simulink model "Vehicle_Radar_Model"  (R2013a)
settings: Solver=ode4  StartTime=0.0  StopTime=100  FixedStep=0.001  MaxStep=0.001  RelTol=1e-3
model workspace (MAT data in the model file):
  m = 1530
  lf = 1.11
  lr = 1.6662
  R_Tire = 0.33
  Iyy_Tire = 0.9
  Pb2Tq_f = 300
  Pb2Tq_r = 150
  Fx_SL = [-1; -0.9; -0.8; -0.7; -0.6; -0.5; -0.4; -0.3; -0.25; -0.2; -0.18; -0.16; -0.14; -0.12; -0.1; -0.08; -0.06; -0.04; -0.02; 0; 0.02; 0.04; 0.06; 0.08; 0.1; 0.12; 0.14; 0.16; 0.18; 0.2; 0.25; 0.3; 0.4; 0.5; 0.6; 0.7; 0.8; 0.9; 1]
  Fx_W = [2105 3995 6120 7900 10100]
  Fx_Data = [-2029.26  -4058.51  -6087.76  -8117.01  -10146.3; -2029.26  -4058.51  -6087.76  -8117.01  -10146.3; -2053.55  -4107.12  -6160.67  -8214.24  -10267.8; -2084.58  -4169.16  -6253.75  -8338.33  -10422.9; -2125.47  -4250.95  -6376.42  -8501.91  -10627.4; -2181.64  -4363.28  -6544.93  -8726.56  -10908.2; -2262.94  -4525.87  -6788.82  -9051.76  -11314.7; -2388.22  -4776.46  -7164.69  -9552.92  -11941.1; -2476.95  -4953.9  -7430.85  -9907.79  -12384.7; -2586.89  -5173.78  -7760.68  -10347.6  -12934.4; -2634.75  -5269.5  -7904.24  -10539  -13173.7; -2680.7  -5361.4  -8042.1  -10722.8  -13403.5; -2717.36  -5434.73  -8152.09  -10869.4  -13586.8; -2729.82  -5459.63  -8189.45  -10919.3  -13649.1; -2689.78  -5379.54  -8069.32  -10759.1  -13448.8; -2548.95  -5097.92  -7646.88  -10195.8  -12744.8; -2240.07  -4480.13  -6720.21  -8960.27  -11200.3; -1701.43  -3402.86  -5104.29  -6805.72  -8507.15; -926.741  -1853.48  -2780.22  -3706.97  -4633.7; 0  0  0  0  0; 926.741  1853.48  2780.22  3706.97  4633.7; 1701.43  3402.86  5104.29  6805.72  8507.15; 2240.07  4480.13  6720.21  8960.27  11200.3; 2548.95  5097.92  7646.88  10195.8  12744.8; 2689.78  5379.54  8069.32  10759.1  13448.8; 2729.82  5459.63  8189.45  10919.3  13649.1; 2717.36  5434.73  8152.09  10869.4  13586.8; 2680.7  5361.4  8042.1  10722.8  13403.5; 2634.75  5269.5  7904.24  10539  13173.7; 2586.89  5173.78  7760.68  10347.6  12934.4; 2476.95  4953.9  7430.85  9907.79  12384.7; 2388.22  4776.46  7164.69  9552.92  11941.1; 2262.94  4525.87  6788.82  9051.76  11314.7; 2181.64  4363.28  6544.93  8726.56  10908.2; 2125.47  4250.95  6376.42  8501.91  10627.4; 2084.58  4169.16  6253.75  8338.33  10422.9; 2053.55  4107.12  6160.67  8214.24  10267.8; 2029.26  4058.51  6087.76  8117.01  10146.3; 2029.26  4058.51  6087.76  8117.01  10146.3]
  g = 9.81
  l = 2.77622
  t2e = 2000
settings Model: Creator=Park  LastModifiedBy=IVDL
settings DataIOCC: LimitDataPoints=off  SignalLoggingSaveFormat=ModelDataLogs
settings OptimizationCC: ExpressionDepthLimit=2147483647
settings DebuggingCC: MultiTaskDSMMsg=warning  MultiTaskCondExecSysMsg=none  FcnCallInpInsideContextMsg=UseLocalSettings  StrictBusMsg=None
settings RTWCC: IncludeERTFirstTime=on
settings GRTTargetCC: CodeReplacementLibrary=None  CombineOutputUpdateFcns=off  CPPClassGenCompliant=on  GRTInterface=on

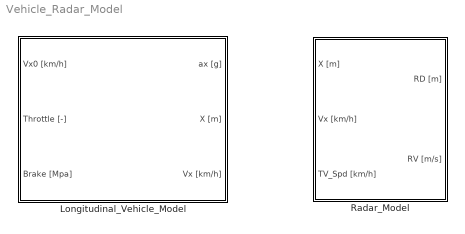
== system Vehicle_Radar_Model ==
  Longitudinal_Vehicle_Model : Subsystem
  Radar_Model : Subsystem

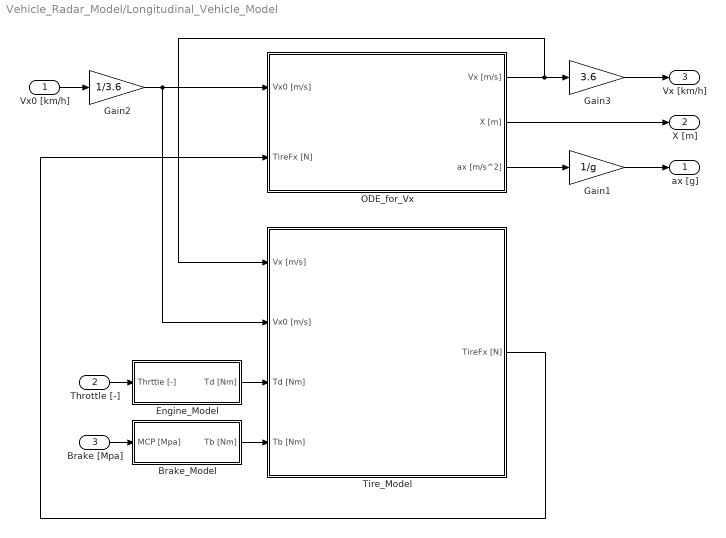
== system Vehicle_Radar_Model/Longitudinal_Vehicle_Model ==
  Vx0 [km/h] : Inport
  Throttle [-] : Inport  Port=2
  Brake [Mpa] : Inport  Port=3
  Brake_Model : Subsystem
  Engine_Model : Subsystem
  Gain1 : Gain  Gain=1/g
  Gain2 : Gain  Gain=1/3.6
  Gain3 : Gain  Gain=3.6
  ODE_for_Vx : Subsystem
  Tire_Model : Subsystem
  ax [g] : Outport
  X [m] : Outport  Port=2
  Vx [km/h] : Outport  Port=3
  wires:
  ODE_for_Vx/2(X [m]) -> X [m]/1
  Vx0 [km/h]/1 -> Gain2/1
  Engine_Model/1(Td [Nm]) -> Tire_Model/3(Td [Nm])
  Brake_Model/1(Tb [Nm]) -> Tire_Model/4(Tb [Nm])
  Brake [Mpa]/1 -> Brake_Model/1(MCP [Mpa])
  Throttle [-]/1 -> Engine_Model/1(Thrttle [-])
  Tire_Model/1(TireFx [N]) -> ODE_for_Vx/2(TireFx [N])
  ODE_for_Vx/3(ax [m/s^2]) -> Gain1/1
  Gain1/1 -> ax [g]/1
  ODE_for_Vx/1(Vx [m/s]) -> Gain3/1, Tire_Model/1(Vx [m/s])
  Gain2/1 -> ODE_for_Vx/1(Vx0 [m/s]), Tire_Model/2(Vx0 [m/s])
  Gain3/1 -> Vx [km/h]/1

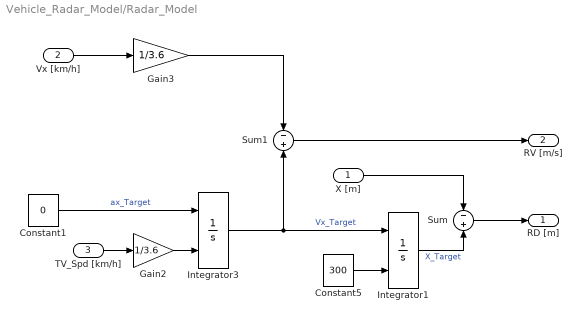
== system Vehicle_Radar_Model/Radar_Model ==
  X [m] : Inport
  Vx [km/h] : Inport  Port=2
  TV_Spd [km/h] : Inport  Port=3
  Constant1 : Constant  Value=0
  Constant5 : Constant  Value=300
  Gain2 : Gain  Gain=1/3.6
  Gain3 : Gain  Gain=1/3.6
  Integrator1 : Integrator  InitialConditionSource=external  InitialCondition=500
  Integrator3 : Integrator  InitialConditionSource=external  InitialCondition=80  LimitOutput=on  LowerSaturationLimit=0
  Sum : Sum  Inputs=-+
  Sum1 : Sum  Inputs=-+
  RD [m] : Outport
  RV [m/s] : Outport  Port=2
  wires:
  TV_Spd [km/h]/1 -> Gain2/1
  Constant1/1 -> Integrator3/1  "ax_Target"
  Integrator3/1 -> Integrator1/1, Sum1/2  "Vx_Target"
  Integrator1/1 -> Sum/2  "X_Target"
  Constant5/1 -> Integrator1/2
  Sum/1 -> RD [m]/1
  X [m]/1 -> Sum/1
  Vx [km/h]/1 -> Gain3/1
  Sum1/1 -> RV [m/s]/1
  Gain2/1 -> Integrator3/2
  Gain3/1 -> Sum1/1

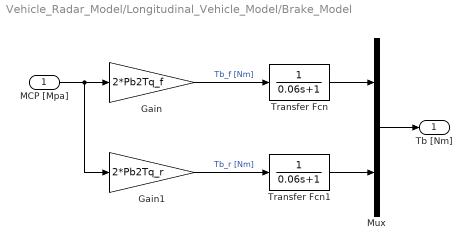
== system Vehicle_Radar_Model/Longitudinal_Vehicle_Model/Brake_Model ==
  MCP [Mpa] : Inport
  Gain : Gain  Gain=2*Pb2Tq_f
  Gain1 : Gain  Gain=2*Pb2Tq_r
  Mux : Mux  Inputs=2
  Transfer Fcn : TransferFcn  Denominator=[0.06 1]
  Transfer Fcn1 : TransferFcn  Denominator=[0.06 1]
  Tb [Nm] : Outport
  wires:
  Gain/1 -> Transfer Fcn/1  "Tb_f [Nm]"
  Gain1/1 -> Transfer Fcn1/1  "Tb_r [Nm]"
  MCP [Mpa]/1 -> Gain1/1, Gain/1
  Mux/1 -> Tb [Nm]/1
  Transfer Fcn/1 -> Mux/1
  Transfer Fcn1/1 -> Mux/2

== system Vehicle_Radar_Model/Longitudinal_Vehicle_Model/Engine_Model ==
  Thrttle [-] : Inport
  Gain : Gain  Gain=t2e
  Transfer Fcn : TransferFcn  Numerator=[100]  Denominator=[1 2*0.5*10 100]
  Td [Nm] : Outport
  wires:
  Thrttle [-]/1 -> Gain/1
  Gain/1 -> Transfer Fcn/1
  Transfer Fcn/1 -> Td [Nm]/1

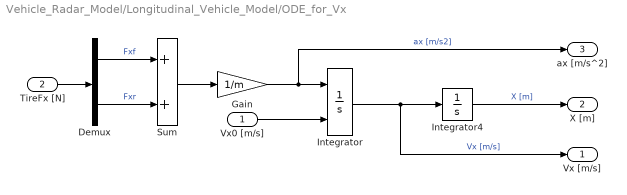
== system Vehicle_Radar_Model/Longitudinal_Vehicle_Model/ODE_for_Vx ==
  Vx0 [m/s] : Inport
  TireFx [N] : Inport  Port=2
  Demux : Demux  Outputs=2
  Gain : Gain  Gain=1/m
  Integrator : Integrator  InitialConditionSource=external
  Integrator4 : Integrator
  Sum : Sum
  Vx [m/s] : Outport
  X [m] : Outport  Port=2
  ax [m/s^2] : Outport  Port=3
  wires:
  Integrator4/1 -> X [m]/1  "X [m]"
  Vx0 [m/s]/1 -> Integrator/2
  Integrator/1 -> Integrator4/1, Vx [m/s]/1  "Vx [m/s]"
  Sum/1 -> Gain/1
  Gain/1 -> Integrator/1, ax [m/s^2]/1  "ax [m/s2]"
  TireFx [N]/1 -> Demux/1
  Demux/1 -> Sum/1  "Fxf"
  Demux/2 -> Sum/2  "Fxr"

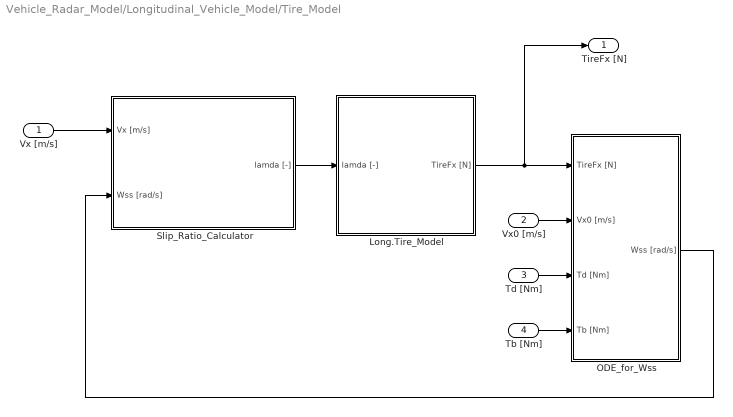
== system Vehicle_Radar_Model/Longitudinal_Vehicle_Model/Tire_Model ==
  Vx [m/s] : Inport
  Vx0 [m/s] : Inport  Port=2
  Td [Nm] : Inport  Port=3
  Tb [Nm] : Inport  Port=4
  Long.Tire_Model : Subsystem
  ODE_for_Wss : Subsystem
  Slip_Ratio_Calculator : Subsystem
  TireFx [N] : Outport
  wires:
  Long.Tire_Model/1(TireFx [N]) -> TireFx [N]/1, ODE_for_Wss/1(TireFx [N])
  Slip_Ratio_Calculator/1(lamda [-]) -> Long.Tire_Model/1(lamda [-])
  Vx [m/s]/1 -> Slip_Ratio_Calculator/1(Vx [m/s])
  Vx0 [m/s]/1 -> ODE_for_Wss/2(Vx0 [m/s])
  Td [Nm]/1 -> ODE_for_Wss/3(Td [Nm])
  Tb [Nm]/1 -> ODE_for_Wss/4(Tb [Nm])
  ODE_for_Wss/1(Wss [rad/s]) -> Slip_Ratio_Calculator/2(Wss [rad/s])

== system Vehicle_Radar_Model/Longitudinal_Vehicle_Model/Tire_Model/Long.Tire_Model ==
  lamda [-] : Inport
  Demux : Demux  Outputs=2
  Fx_f_Calculator : Subsystem
  Fx_r_Calculator : Subsystem
  Mux : Mux  Inputs=2
  TireFx [N] : Outport
  wires:
  lamda [-]/1 -> Demux/1
  Demux/1 -> Fx_f_Calculator/1(lamda_f [-])
  Demux/2 -> Fx_r_Calculator/1(lamda_r [-])
  Fx_f_Calculator/1(TireFx _f [N]) -> Mux/1
  Fx_r_Calculator/1(TireFx _r [N]) -> Mux/2
  Mux/1 -> TireFx [N]/1

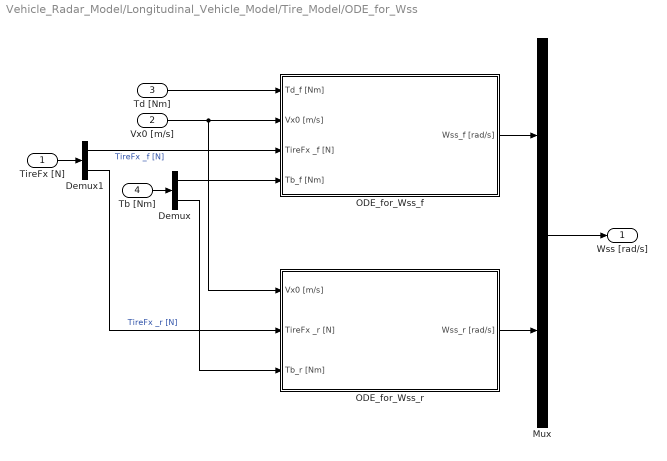
== system Vehicle_Radar_Model/Longitudinal_Vehicle_Model/Tire_Model/ODE_for_Wss ==
  TireFx [N] : Inport
  Vx0 [m/s] : Inport  Port=2
  Td [Nm] : Inport  Port=3
  Tb [Nm] : Inport  Port=4
  Demux : Demux  Outputs=2
  Demux1 : Demux  Outputs=2
  Mux : Mux  Inputs=2
  ODE_for_Wss_f : Subsystem
  ODE_for_Wss_r : Subsystem
  Wss [rad/s] : Outport
  wires:
  Demux1/1 -> ODE_for_Wss_f/3(TireFx _f [N])  "TireFx _f [N]"
  Td [Nm]/1 -> ODE_for_Wss_f/1(Td_f [Nm])
  Vx0 [m/s]/1 -> ODE_for_Wss_r/1(Vx0 [m/s]), ODE_for_Wss_f/2(Vx0 [m/s])
  Tb [Nm]/1 -> Demux/1
  Demux/1 -> ODE_for_Wss_f/4(Tb_f [Nm])
  Demux/2 -> ODE_for_Wss_r/3(Tb_r [Nm])
  TireFx [N]/1 -> Demux1/1
  Demux1/2 -> ODE_for_Wss_r/2(TireFx _r [N])  "TireFx _r [N]"
  ODE_for_Wss_f/1(Wss_f [rad/s]) -> Mux/1
  ODE_for_Wss_r/1(Wss_r [rad/s]) -> Mux/2
  Mux/1 -> Wss [rad/s]/1

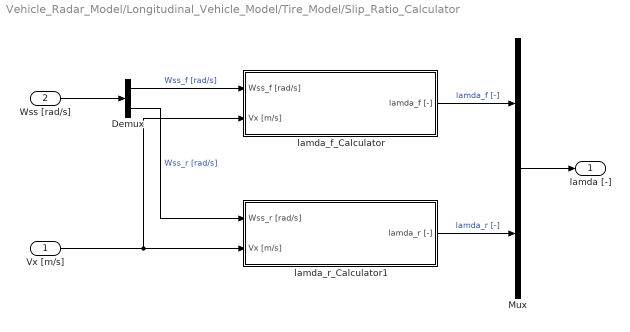
== system Vehicle_Radar_Model/Longitudinal_Vehicle_Model/Tire_Model/Slip_Ratio_Calculator ==
  Vx [m/s] : Inport
  Wss [rad/s] : Inport  Port=2
  Demux : Demux  Outputs=2
  Mux : Mux  Inputs=2
  lamda_f_Calculator : Subsystem
  lamda_r_Calculator1 : Subsystem
  lamda [-] : Outport
  wires:
  Vx [m/s]/1 -> lamda_f_Calculator/2(Vx [m/s]), lamda_r_Calculator1/2(Vx [m/s])
  lamda_f_Calculator/1(lamda_f [-]) -> Mux/1  "lamda_f [-]"
  lamda_r_Calculator1/1(lamda_r [-]) -> Mux/2  "lamda_r [-]"
  Mux/1 -> lamda [-]/1
  Wss [rad/s]/1 -> Demux/1
  Demux/1 -> lamda_f_Calculator/1(Wss_f [rad/s])  "Wss_f [rad/s]"
  Demux/2 -> lamda_r_Calculator1/1(Wss_r [rad/s])  "Wss_r [rad/s]"

== system Vehicle_Radar_Model/Longitudinal_Vehicle_Model/Tire_Model/Long.Tire_Model/Fx_f_Calculator ==
  lamda_f [-] : Inport
  Constant : Constant  Value=m*9.81
  Fx_Table_fl : Lookup2D  RowIndex=Fx_SL  ColumnIndex=Fx_W  Table=Fx_Data  SaturateOnIntegerOverflow=on
  Gain : Gain  Gain=lr / (lf+lr)
  Gain1 : Gain  Gain=2
  Gain4 : Gain  Gain=0.5
  TireFx _f [N] : Outport
  wires:
  Gain1/1 -> TireFx _f [N]/1
  lamda_f [-]/1 -> Fx_Table_fl/1
  Constant/1 -> Gain/1
  Gain/1 -> Gain4/1
  Gain4/1 -> Fx_Table_fl/2  "Wf [N]"
  Fx_Table_fl/1 -> Gain1/1

== system Vehicle_Radar_Model/Longitudinal_Vehicle_Model/Tire_Model/Long.Tire_Model/Fx_r_Calculator ==
  lamda_r [-] : Inport
  Constant1 : Constant  Value=m*9.81
  Fx_Table_fl1 : Lookup2D  RowIndex=Fx_SL  ColumnIndex=Fx_W  Table=Fx_Data  SaturateOnIntegerOverflow=on
  Gain2 : Gain  Gain=lf / (lf+lr)
  Gain3 : Gain  Gain=2
  Gain5 : Gain  Gain=0.5
  TireFx _r [N] : Outport
  wires:
  lamda_r [-]/1 -> Fx_Table_fl1/1
  Constant1/1 -> Gain2/1
  Fx_Table_fl1/1 -> Gain3/1
  Gain2/1 -> Gain5/1
  Gain5/1 -> Fx_Table_fl1/2  "Wr [N]"
  Gain3/1 -> TireFx _r [N]/1

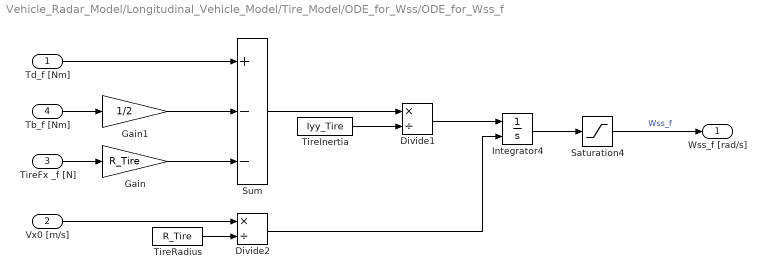
== system Vehicle_Radar_Model/Longitudinal_Vehicle_Model/Tire_Model/ODE_for_Wss/ODE_for_Wss_f ==
  Td_f [Nm] : Inport
  Vx0 [m/s] : Inport  Port=2
  TireFx _f [N] : Inport  Port=3
  Tb_f [Nm] : Inport  Port=4
  Divide1 : Product  Inputs=*/
  Divide2 : Product  Inputs=*/
  Gain : Gain  Gain=R_Tire
  Gain1 : Gain  Gain=1/2
  Integrator4 : Integrator  InitialConditionSource=external
  Saturation4 : Saturate  UpperLimit=255  LowerLimit=0
  Sum : Sum  Inputs=+--
  TireInertia : Constant  Value=Iyy_Tire
  TireRadius : Constant  Value=R_Tire
  Wss_f [rad/s] : Outport
  wires:
  Gain/1 -> Sum/3
  Td_f [Nm]/1 -> Sum/1
  Tb_f [Nm]/1 -> Gain1/1
  TireFx _f [N]/1 -> Gain/1
  Sum/1 -> Divide1/1
  TireInertia/1 -> Divide1/2
  Divide1/1 -> Integrator4/1
  TireRadius/1 -> Divide2/2
  Vx0 [m/s]/1 -> Divide2/1
  Divide2/1 -> Integrator4/2
  Integrator4/1 -> Saturation4/1
  Saturation4/1 -> Wss_f [rad/s]/1  "Wss_f"
  Gain1/1 -> Sum/2

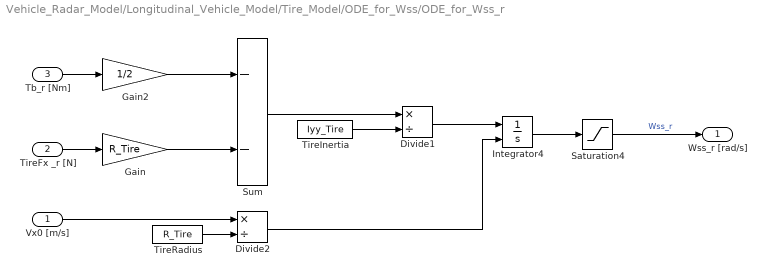
== system Vehicle_Radar_Model/Longitudinal_Vehicle_Model/Tire_Model/ODE_for_Wss/ODE_for_Wss_r ==
  Vx0 [m/s] : Inport
  TireFx _r [N] : Inport  Port=2
  Tb_r [Nm] : Inport  Port=3
  Divide1 : Product  Inputs=*/
  Divide2 : Product  Inputs=*/
  Gain : Gain  Gain=R_Tire
  Gain2 : Gain  Gain=1/2
  Integrator4 : Integrator  InitialConditionSource=external
  Saturation4 : Saturate  UpperLimit=255  LowerLimit=0
  Sum : Sum  Inputs=--
  TireInertia : Constant  Value=Iyy_Tire
  TireRadius : Constant  Value=R_Tire
  Wss_r [rad/s] : Outport
  wires:
  Saturation4/1 -> Wss_r [rad/s]/1  "Wss_r"
  Integrator4/1 -> Saturation4/1
  Divide2/1 -> Integrator4/2
  Vx0 [m/s]/1 -> Divide2/1
  TireRadius/1 -> Divide2/2
  Divide1/1 -> Integrator4/1
  TireInertia/1 -> Divide1/2
  Sum/1 -> Divide1/1
  TireFx _r [N]/1 -> Gain/1
  Tb_r [Nm]/1 -> Gain2/1
  Gain/1 -> Sum/2
  Gain2/1 -> Sum/1

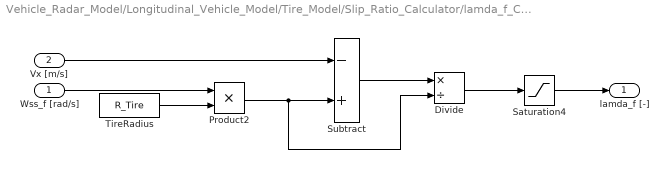
== system Vehicle_Radar_Model/Longitudinal_Vehicle_Model/Tire_Model/Slip_Ratio_Calculator/lamda_f_Calculator ==
  Wss_f [rad/s] : Inport
  Vx [m/s] : Inport  Port=2
  Divide : Product  Inputs=*/
  Product2 : Product  RndMeth=Zero
  Saturation4 : Saturate  UpperLimit=1  LowerLimit=-1
  Subtract : Sum  Inputs=-+
  TireRadius : Constant  Value=R_Tire
  lamda_f [-] : Outport
  wires:
  Vx [m/s]/1 -> Subtract/1
  Wss_f [rad/s]/1 -> Product2/1
  TireRadius/1 -> Product2/2
  Product2/1 -> Subtract/2, Divide/2
  Subtract/1 -> Divide/1
  Divide/1 -> Saturation4/1
  Saturation4/1 -> lamda_f [-]/1

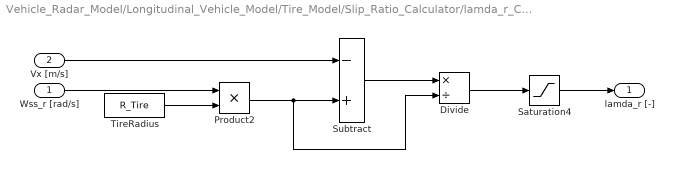
== system Vehicle_Radar_Model/Longitudinal_Vehicle_Model/Tire_Model/Slip_Ratio_Calculator/lamda_r_Calculator1 ==
  Wss_r [rad/s] : Inport
  Vx [m/s] : Inport  Port=2
  Divide : Product  Inputs=*/
  Product2 : Product  RndMeth=Zero
  Saturation4 : Saturate  UpperLimit=1  LowerLimit=-1
  Subtract : Sum  Inputs=-+
  TireRadius : Constant  Value=R_Tire
  lamda_r [-] : Outport
  wires:
  Saturation4/1 -> lamda_r [-]/1
  Divide/1 -> Saturation4/1
  Subtract/1 -> Divide/1
  Product2/1 -> Divide/2, Subtract/2
  TireRadius/1 -> Product2/2
  Wss_r [rad/s]/1 -> Product2/1
  Vx [m/s]/1 -> Subtract/1
